simulink model "openloop_response"  (R2021a)
settings: Solver=ode15s  StartTime=0.0  StopTime=20  RelTol=1e-7  AbsTol=1e-7  EnableMultiTasking=on
InitFcn:
  | datacstr
values from neighbouring files (symbols this model uses):
  c_bar = 0.5    [main.m]
  T_bar = 350    [main.m]
settings Model: ExtModeTrigMode=oneshot  ExtModeArmWhenConnect=off  Creator=scattolini  LastModifiedBy=fabio
settings SolverCC: AutoScaleAbsTol=off  AlgebraicLoopSolver=TrustRegion
settings DataIOCC: SaveFormat=Array  SignalLoggingSaveFormat=ModelDataLogs  ReturnWorkspaceOutputs=off  SignalLoggingName=sigsOut
settings OptimizationCC: BlockReduction=off  BooleanDataType=off  DefaultParameterBehavior=Inlined  BufferReuse=off  ExpressionDepthLimit=2147483647  InitFltsAndDblsToZero=on  LifeSpan=inf
settings DebuggingCC: SaveWithParameterizedLinksMsg=none  UnderspecifiedInitializationDetection=Classic  MergeDetectMultiDrivingBlocksExec=none  SignalResolutionControl=TryResolveAllWithWarning  MultiTaskDSMMsg=warning  MultiTaskCondExecSysMsg=none  FcnCallInpInsideContextMsg=warning  StateNameClashWarn=warning  SFUnexpectedBacktrackingDiag=warning  SFNoUnconditionalDefaultTransitionDiag=warning  SFExecutionAtInitializationDiag=none  SFMachineParentedDataDiag=warning  ArithmeticOperatorsInVariantConditions=warning
settings HardwareCC: ProdBitPerPointer=32  ProdBitPerSizeT=32  ProdBitPerPtrDiffT=32  ProdLargestAtomicFloat=None  ProdIntDivRoundTo=Undefined  ProdEndianess=Unspecified  ProdWordSize=32  ProdHWDeviceType=32-bit Generic  TargetUnknown=on
settings ModelReferenceCC: PropagateSignalLabelsOutOfModel=off
settings SFSimCC: SimUseLocalCustomCode=off  CustomCodeUndefinedFunction=UseInterfaceOnly
settings RTWCC: Description=Generic Real-Time Target  RTWUseLocalCustomCode=off
settings CodeAppCC: StateflowObjectComments=on
settings GRTTargetCC: TargetFcnLib=ansi_tfl_tmw.mat  TargetLangStandard=C89/C90 (ANSI)  CombineOutputUpdateFcns=off  GRTInterface=on
settings ConfigComp: CovMetricSettings=dw  CovSaveCumulativeToWorkspaceVar=on  CovSaveSingleToWorkspaceVar=on  CovExternalEMLEnable=off  CovSFcnEnable=off

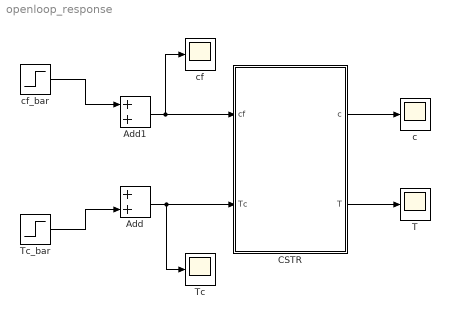
== system openloop_response ==
  Add : Sum
  Add1 : Sum
  CSTR : Subsystem
      settings: AttributesFormatString=%<Description>
  T : Scope
  Tc : Scope
  Tc_bar : Step  Time=0  Before=300  After=300  SampleTime=0
  c : Scope
  cf : Scope
  cf_bar : Step  Time=0  Before=1  SampleTime=0
  wires:
  CSTR/2(T) -> T/1
  Add/1 -> Tc/1, CSTR/2(Tc)
  Add1/1 -> cf/1, CSTR/1(cf)
  Tc_bar/1 -> Add/2
  cf_bar/1 -> Add1/1
  CSTR/1(c) -> c/1

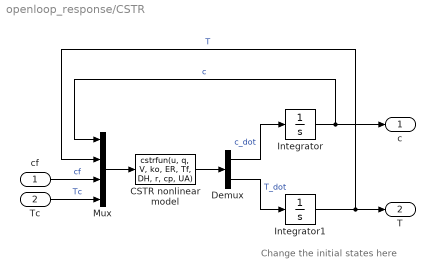
== system openloop_response/CSTR ==
  note: Change the initial
      | states here
  cf : Inport
  Tc : Inport  Port=2
  CSTR nonlinear model : MATLABFcn  MATLABFcn=cstrfun(u, q, V, ko, ER, Tf, DH, r, cp, UA)  OutputDimensions=2
  Demux : Demux  Outputs=2
      settings: DisplayOption=none
  Integrator : Integrator  InitialCondition=c_bar
  Integrator1 : Integrator  InitialCondition=T_bar
  Mux : Mux
  c : Outport
  T : Outport  Port=2
  wires:
  Mux/1 -> CSTR nonlinear model/1
  CSTR nonlinear model/1 -> Demux/1
  Demux/1 -> Integrator/1  "c_dot"
  Demux/2 -> Integrator1/1  "T_dot"
  Integrator1/1 -> Mux/2, T/1  "T"
  Integrator/1 -> c/1, Mux/1  "c"
  cf/1 -> Mux/3  "cf"
  Tc/1 -> Mux/4  "Tc"
